simulink model "Lateral_Vehicle_dyn_TV_Nonlin_Long_Control_TV_GPC_SV1"  (R2019b)
settings: Solver=FixedStepAuto  StartTime=0.0  StopTime=20  FixedStep=1.e-4  RelTol=1e-3
values from neighbouring files (symbols this model uses):
  H = zeros (rB*n, cB*n)    [eq_linearise_Discrete_MPC.m]
  l = 3    [eq_linearise_Discrete_MPC.m]
  m = 1500    [eq_linearise_Discrete_MPC.m]
  P = zeros (rA*n, cA)    [eq_linearise_Discrete_MPC.m]
  Q = diag (q)    [eq_linearise_Discrete_MPC.m]
  R = diag (r)    [eq_linearise_Discrete_MPC.m]
  rw = 0.28    [eq_linearise_Discrete_MPC.m]
undefined symbols (not defined in the file or in its folder): sigbuilder_block
libraries: simulink x1
settings Model: Creator=admin  LastModifiedBy=admin

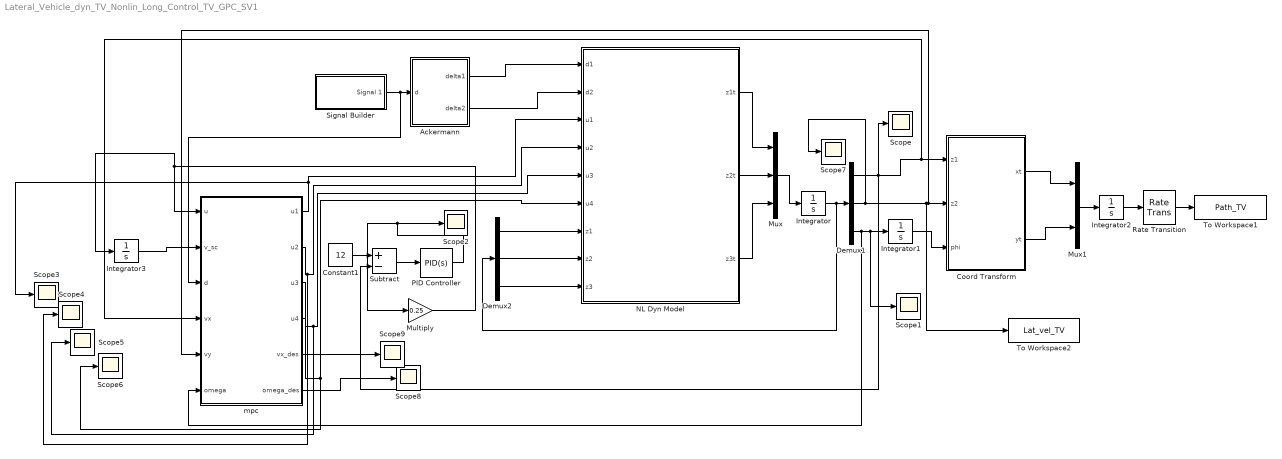
== system Lateral_Vehicle_dyn_TV_Nonlin_Long_Control_TV_GPC_SV1 ==
  Ackermann : MATLAB Function  TreatAsAtomicUnit=on
  Constant1 : Constant  Value=12
  Coord Transform : MATLAB Function  TreatAsAtomicUnit=on
  Demux1 : Demux  Outputs=3
  Demux2 : Demux  Outputs=3
  Integrator : Integrator  InitialCondition=[4 0 0]
  Integrator1 : Integrator  InitialCondition=[0]
  Integrator2 : Integrator  InitialCondition=[0 0]
  Integrator3 : Integrator  InitialCondition=[0]
  Multiply : Gain  Gain=0.25
  Mux : Mux  Inputs=3
  Mux1 : Mux  Inputs=2
  NL Dyn Model : MATLAB Function  TreatAsAtomicUnit=on
  PID Controller : simulink/Continuous/PID Controller  Controller=PID  Form=Parallel  TimeDomain=Continuous-time  SampleTime=-1  IntegratorMethod=Forward Euler  FilterMethod=Forward Euler  ControllerParametersSource=internal  P=150  I=0  D=0  UseFilter=on  N=100  TunerSelectOption=Transfer Function Based (PID Tuner App)  InitialConditionSource=internal  InitialConditionForIntegrator=0  InitialConditionForFilter=0  DifferentiatorICPrevScaledInput=0  ExternalReset=none  TrackingMode=off  Kt=1  LimitOutput=off  UpperSaturationLimit=inf  LowerSaturationLimit=-inf  LinearizeAsGain=on  AntiWindupMode=none  Kb=1  POutMin=[]  POutMax=[]  IOutMin=[]  IOutMax=[]  DOutMin=[]  DOutMax=[]  NOutMin=[]  NOutMax=[]  SumOutMin=[]  SumOutMax=[]  SaturationOutMin=[]  SaturationOutMax=[]  PParamMin=[]  PParamMax=[]  IParamMin=[]  IParamMax=[]  DParamMin=[]  DParamMax=[]  NParamMin=[]  NParamMax=[]  KbParamMin=[]  KbParamMax=[]  KtParamMin=[]  KtParamMax=[]  KbOutMin=[]  KbOutMax=[]  KtOutMin=[]  KtOutMax=[]  IntegratorOutMin=[]  IntegratorOutMax=[]  FilterOutMin=[]  FilterOutMax=[]  SumI1OutMin=[]  SumI1OutMax=[]  SumI2OutMin=[]  SumI2OutMax=[]  SumI3OutMin=[]  SumI3OutMax=[]  SumI4OutMin=[]  SumI4OutMax=[]  SumDOutMin=[]  SumDOutMax=[]  DifferentiatorOutMin=[]  DifferentiatorOutMax=[]  FilterDiffOutCoefMin=[]  FilterDiffOutCoefMax=[]  ReciprocalOutMin=[]  ReciprocalOutMax=[]  SumDenOutMin=[]  SumDenOutMax=[]  SumNumOutMin=[]  SumNumOutMax=[]  DivideOutMin=[]  DivideOutMax=[]  IntegratorContinuousStateAttributes=''  IntegratorStateMustResolveToSignalObject=off  IntegratorRTWStateStorageClass=Auto  FilterContinuousStateAttributes=''  FilterStateMustResolveToSignalObject=off  FilterRTWStateStorageClass=Auto  ParallelPVariant=InternalParameters  IdealPVariant=Disabled  IVariant=InternalParameters  DVariant=InternalParameters  IntegratorVariant=Continuous  SatVariant=Disabled  AWVariant=Passthrough  PCopyVariant=Disabled  TRVariant=Disabled  FdbkBlocksVariant=Forward  IdealPFdbkVariant=Disabled  SatFdbkVariant=Disabled  DerivativeFilterVariant=ContFilter  NVariant=InternalParameters  NCopyVariant=Disabled  FilterICVariant=InternalICsFilter  IntegratorICVariant=InternalICs  ExternalResetVariant=Disabled  TRSumVariant=Passthrough  SumFdbkVariant=Disabled  SumVariant=Sum_PID
  Rate Transition : RateTransition  OutPortSampleTime=0.01
  Scope{,1..9} (10 alike) : Scope
  Signal Builder : Subsystem  Tag=STV Subsys  LoadFcn=sigbuilder_block('load');  StartFcn=sigbuilder_block('start');  StopFcn=sigbuilder_block('stop');  ClipboardFcn=sigbuilder_block('clipboard');  mask(Sigbuilder block){tuvar=[0:10]}
      mask help: Simulink:masks:SigbuilderBlock_MD
      mask init:
      | if ~strcmp(get_param(bdroot(gcbh),'SimulationStatus'),'stopped') tuvar = sigbuilder_block('maskInit'); end
      settings: CopyFcn=sigbuilder_block('copy');  DeleteFcn=sigbuilder_block('delete');  ModelCloseFcn=sigbuilder_block('modelClose');  PreSaveFcn=sigbuilder_block('preSave');  PauseFcn=sigbuilder_block('pause');  ContinueFcn=sigbuilder_block('continue');  NameChangeFcn=sigbuilder_block('namechange');  OpenFcn=sigbuilder_block('open',[437.6 85.5 550.4 426.75 ]);  CloseFcn=sigbuilder_block('close');
      mask Display: plot(0, 0, 100, 100,[2, 2, 32, 32, 2], [68, 8, 8, 68, 68],[32, 2], [38, 38], [32, 19, 2],[53, 60, 44], [32, 17, 17, 2],[16, 16, 31, 31]);txt = getActiveGroup(gcbh);text(2, 100, txt,'verticalAlignment', 'top');
  Subtract : Sum  Inputs=+-
  To Workspace1 : ToWorkspace  VariableName=Path_TV  SaveFormat=Timeseries  SampleTime=-1
  To Workspace2 : ToWorkspace  VariableName=Lat_vel_TV  SaveFormat=Timeseries  SampleTime=-1
  "mpc " : MATLAB Function  TreatAsAtomicUnit=on
  wires:
  NL Dyn Model/1(z1t) -> Mux/1
  NL Dyn Model/2(z2t) -> Mux/2
  NL Dyn Model/3(z3t) -> Mux/3
  Mux/1 -> Integrator/1
  Integrator/1 -> Demux2/1, Demux1/1
  Demux1/2 -> Scope7/1, To Workspace2/1, "mpc "/5(vy), Coord Transform/2(z2)
  Demux1/3 -> "mpc "/6(omega), Scope1/1, Integrator1/1
  Integrator1/1 -> Coord Transform/3(phi)
  Coord Transform/1(xt) -> Mux1/1
  Coord Transform/2(yt) -> Mux1/2
  Mux1/1 -> Integrator2/1
  Integrator2/1 -> Rate Transition/1
  Rate Transition/1 -> To Workspace1/1
  Ackermann/1(delta1) -> NL Dyn Model/1(d1)
  Ackermann/2(delta2) -> NL Dyn Model/2(d2)
  Demux2/1 -> NL Dyn Model/7(z1)
  Demux2/2 -> NL Dyn Model/8(z2)
  Demux2/3 -> NL Dyn Model/9(z3)
  PID Controller/1 -> Scope2/1, Multiply/1
  Signal Builder/1(Signal 1) -> "mpc "/3(d), Ackermann/1(d)
  Constant1/1 -> Subtract/1
  Demux1/1 -> Subtract/2, Scope/1, "mpc "/4(vx), Coord Transform/1(z1)
  Subtract/1 -> PID Controller/1
  Multiply/1 -> Integrator3/1, "mpc "/1(u)
  Integrator3/1 -> "mpc "/2(v_sc)
  "mpc "/1(u1) -> Scope3/1, NL Dyn Model/3(u1)
  "mpc "/2(u2) -> Scope4/1, NL Dyn Model/4(u2)
  "mpc "/3(u3) -> Scope5/1, NL Dyn Model/5(u3)
  "mpc "/4(u4) -> Scope6/1, NL Dyn Model/6(u4)
  "mpc "/5(vx_des) -> Scope9/1
  "mpc "/6(omega_des) -> Scope8/1

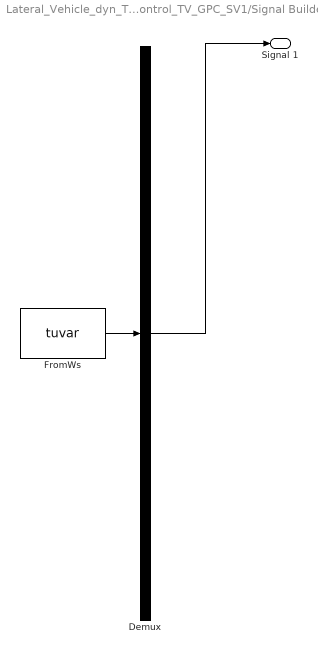
== system Lateral_Vehicle_dyn_TV_Nonlin_Long_Control_TV_GPC_SV1/Signal Builder ==
  Demux : Demux  Tag=STV Demux  Outputs=1
  FromWs : FromWorkspace  Tag=STV FromWs  VariableName=tuvar  SampleTime=0
      SigBuilderData=|
      | common.afterFinalStr = 'Extrapolate'
      | common.sampleTime = 0
      | dataSet.timeRange = [0 10]
      | dataSet.name = 'Group 1'
      | sbobj.Groups.Name = 'Group 1'
      | sbobj.Groups.Signals.Name = 'Signal 1'
      | sbobj.Groups.Signals.XData = [0 0.5 10]
      | sbobj.Groups.Signals.YData = [0 0.4 0.4]
  Signal 1 : Outport  Tag=STV Outport
  wires:
  Demux/1 -> Signal 1/1
  FromWs/1 -> Demux/1

== matlab function Lateral_Vehicle_dyn_TV_Nonlin_Long_Control_TV_GPC_SV1/Coord Transform ==
  data: z1 input; z2 input; phi input; xt output; yt output
function [ xt , yt ] = dyn_model ( z1 , z2 , phi )

xt=z1*cos(phi) - z2*sin(phi);
yt=z1*sin(phi) + z2*cos(phi);

== matlab function Lateral_Vehicle_dyn_TV_Nonlin_Long_Control_TV_GPC_SV1/NL Dyn Model ==
  data: d1 input; z1t output; d2 input; u1 input; u2 input; u3 input; u4 input; z1 input; z2 input; z3 input; z2t output; z3t output
function [ z1t , z2t , z3t ] = dyn_model ( d1 , d2 , u1 , u2 , u3 , u4 , z1 , z2 , z3 )

% parameter declaration
m = 1500; g = 9.81; rw = 0.28; x1 = 1.3; x2 = 1.3;
x3 = -1.7; x4 = -1.7; y1 = 0.8; y2 = -0.8; y3 = 0.8;
y4 = -0.8; Izz = 2000; d3 = 0; d4 = 0;

% calculating reaction forces
Fz12 = 0.5* m * g *( abs ( x3 ) /( x1 + abs ( x3 ) ) ) ;
Fz34 = 0.5* m * g *( x1 /( x1 + abs ( x3 ) ) ) ;
% calculating longitudinal forces
F1t = u1 / rw ; F2t = u2 / rw ; F3t = u3 / rw ; F4t = u4 / rw ;
% calculating lateral forces
F1s = Fz12 * tyre ( d1 , x1 , y1 , z1 , z2 , z3 ) ;
F2s = Fz12 * tyre ( d2 , x2 , y2 , z1 , z2 , z3 ) ;
F3s = Fz34 * tyre ( d3 , x3 , y3 , z1 , z2 , z3 ) ;
F4s = Fz34 * tyre ( d4 , x4 , y4 , z1 , z2 , z3 ) ;

% dynamic model
z1t = (1/ m ) *( F1t * cos ( d1 ) - F1s * sin ( d1 ) + F2t * cos ( d2 ) - F2s * sin ( d2 ) + F3t + F4t + m * z2 * z3 ) ;
z2t = (1/ m ) *( F1t * sin ( d1 ) + F1s * cos ( d1 ) + F2t * sin ( d2 ) + F2s * cos ( d2 ) + F3s + F4s - m * z1 * z3 ) ;
z3t = (1/ Izz ) *( x1 *( F1t * sin ( d1 ) + F1s * cos ( d1 ) )...
 - y1 *( F1t * cos ( d1 ) - F1s * sin ( d1 ) ) + x2 *( F2t * sin ( d2 )...
 + F2s * cos ( d2 ) ) - y2 *( F2t * cos ( d2 ) - F2s * sin ( d2 ) )...
 + x3 * F3s - y3 * F3t + x4 * F4s - y4 * F4t ) ;

% function computing normalized tyre lateral force
function mu = tyre (d ,x ,y , z1 , z2 , z3 )
alpha_p = 6* pi /180; % peak alpha value
mu_p = 0.9; % peak mu value
alpha = d - atan (( z2 + z3 * x ) /( z1 - z3 * y ) ) ;
mu = ((2* alpha_p * mu_p ) /( alpha_p ^2 + alpha ^2) ) * alpha ;

== matlab function Lateral_Vehicle_dyn_TV_Nonlin_Long_Control_TV_GPC_SV1/Ackermann ==
  data: d input; delta1 output; delta2 output
function [delta1 , delta2 ] = ack(d)
% individual wheel coordinates from center of gravity
y1 = 0.8; y2 = -0.8; x2 = 1.3; x3 = -1.7;
w = (y1 + abs(y2)); % axle track
l = (x2 + abs(x3)); % wheelbase
delta1 = acot (cot (d) - w /(2* l));
delta2 = acot (cot (d) + w /(2* l));

== matlab function Lateral_Vehicle_dyn_TV_Nonlin_Long_Control_TV_GPC_SV1/mpc  ==
  data: u input; u1 output; u2 output; v_sc input; d input; vx input; vy input; omega input; u3 output; u4 output; m parameter; rw parameter; P parameter; Q parameter; H parameter; R parameter; l parameter; vx_des output; omega_des output
function [u1 ,u2 ,u3 ,u4,vx_des,omega_des] = mpc(u,v_sc ,d,vx ,vy , omega,  m, rw, P, Q, H, R, l) %sys ,wgt ,
% deviation from desired state
vx_des = vx + v_sc /( m*rw);
vy_des = 0;
omega_des = vx*tan(d);
% omega_des = vx*tan(d)/l;
x_k = [vx - vx_des ; vy - vy_des ; omega - omega_des ];

% control law
% H = sys.H; P = sys.P; Q = wgt.Q; R = wgt.R;
u_k = -(H'*Q*H + R)\(H'*Q*P*x_k );
u1 = u+u_k (1) ;
u2 = u+u_k (2) ;
u3 = u+u_k (3) ;
u4 = u+u_k (4) ;

return
